simulink model "critical_k"  (R2021a)
settings: Solver=VariableStepAuto  StartTime=0.0  StopTime=20.0  RelTol=1e-3
values from neighbouring files (symbols this model uses):
  a21 = -2*(k+K)/(2*Mt+9*m)    (= -2436.05359318)    [parameters_initialization.m]
  a22 = -2*(b+Bp)/(2*Mt+9*m)    (= -0.219244823386)    [parameters_initialization.m]
  a23 = 2*Ap/(2*Mt+9*m)    (= 1.70523751523e-05)    [parameters_initialization.m]
  a24 = 2*k/(2*Mt+9*m)    (= 2436.05359318)    [parameters_initialization.m]
  a25 = 2*b/(2*Mt+9*m)    (= 0.182704019488)    [parameters_initialization.m]
  a32 = -Ap*4*Be/Vt    (= -18200000000)    [parameters_initialization.m]
  a33 = -4*Be*(Kc+Ctp)/Vt    (= -2.73)    [parameters_initialization.m]
  a51 = k*6/(7*m)    (= 9523.80952381)    [parameters_initialization.m]
  a52 = b*6/(7*m)    (= 0.714285714286)    [parameters_initialization.m]
  a54 = -k*6/(7*m)    (= -9523.80952381)    [parameters_initialization.m]
  a55 = -b*6/(7*m)    (= -0.714285714286)    [parameters_initialization.m]
  b31 = Kq*Kt*4*Be/(Vt*R*r*Kf)    (= 176800000)    [parameters_initialization.m]
  h51 = (6/7)*g    (= 8.40857142857)    [parameters_initialization.m]
settings Model: Creator=st190427d  LastModifiedBy=st190427d
settings SolverCC: AlgebraicLoopSolver=TrustRegion
settings DataIOCC: ReturnWorkspaceOutputs=off
settings DebuggingCC: SFMachineParentedDataDiag=warning  ArithmeticOperatorsInVariantConditions=warning
settings SFSimCC: SimUseLocalCustomCode=off  CustomCodeUndefinedFunction=UseInterfaceOnly
settings RTWCC: RTWUseLocalCustomCode=off

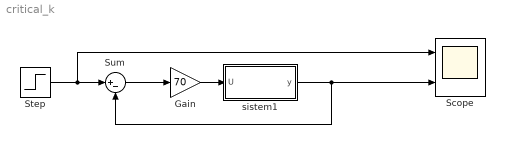
== system critical_k ==
  Gain : Gain  Gain=70
  Scope : Scope  NumInputPorts=2
  Step : Step  After=0.5  SampleTime=0
  Sum : Sum  Inputs=|+-
  sistem1 : Subsystem
  wires:
  Step/1 -> Scope/1, Sum/1
  Sum/1 -> Gain/1
  Gain/1 -> sistem1/1(U)
  sistem1/1(y) -> Scope/2, Sum/2

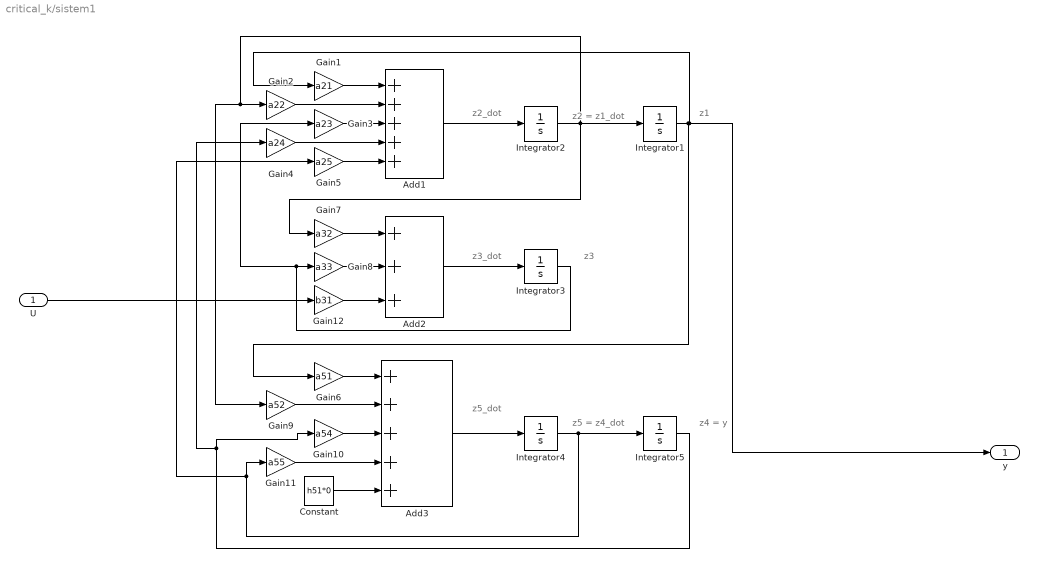
== system critical_k/sistem1 ==
  note: z1
  note: z2 = z1_dot
  note: z2_dot
  note: z3_dot
  note: z3
  note: z4 = y
  note: z5 = z4_dot
  note: z5_dot
  U : Inport
  Add1 : Sum  Inputs=+++++
  Add2 : Sum  Inputs=+++
  Add3 : Sum  Inputs=+++++
  Constant : Constant  Value=h51*0
  Gain1 : Gain  Gain=a21
  Gain10 : Gain  Gain=a54
  Gain11 : Gain  Gain=a55
  Gain12 : Gain  Gain=b31
  Gain2 : Gain  Gain=a22
  Gain3 : Gain  Gain=a23
  Gain4 : Gain  Gain=a24
  Gain5 : Gain  Gain=a25
  Gain6 : Gain  Gain=a51
  Gain7 : Gain  Gain=a32
  Gain8 : Gain  Gain=a33
  Gain9 : Gain  Gain=a52
  Integrator{1..5} (5 alike) : Integrator
  y : Outport  VectorParamsAs1DForOutWhenUnconnected=off
  wires:
  Gain7/1 -> Add2/1
  Add1/1 -> Integrator2/1
  Gain3/1 -> Add1/3
  Add2/1 -> Integrator3/1
  Gain1/1 -> Add1/1
  Integrator1/1 -> y/1, Gain1/1, Gain6/1
  Gain6/1 -> Add3/1
  Integrator3/1 -> Gain3/1, Gain8/1
  Add3/1 -> Integrator4/1
  Gain12/1 -> Add2/3
  Integrator4/1 -> Gain5/1, Gain11/1, Integrator5/1
  Integrator5/1 -> Gain4/1, Gain10/1
  Gain5/1 -> Add1/5
  Gain2/1 -> Add1/2
  Gain11/1 -> Add3/4
  U/1 -> Gain12/1
  Integrator2/1 -> Gain7/1, Gain9/1, Gain2/1, Integrator1/1
  Gain9/1 -> Add3/2
  Gain10/1 -> Add3/3
  Gain8/1 -> Add2/2
  Gain4/1 -> Add1/4
  Constant/1 -> Add3/5
